simulink model "tfs"  (R2017b)
settings: Solver=FixedStepAuto  StartTime=0.0  StopTime=6  FixedStep=T  RelTol=1e-3  EnableMultiTasking=on
values from neighbouring files (symbols this model uses):
  d = [1 -2.638 2.284 -0.6455]    [EJECUTABLE.m]
  n = [0.01584 -0.03175 0.01594]    [EJECUTABLE.m]
undefined symbols (not defined in the file or in its folder): Controlador
settings Model: Creator=camal  LastModifiedBy=camal

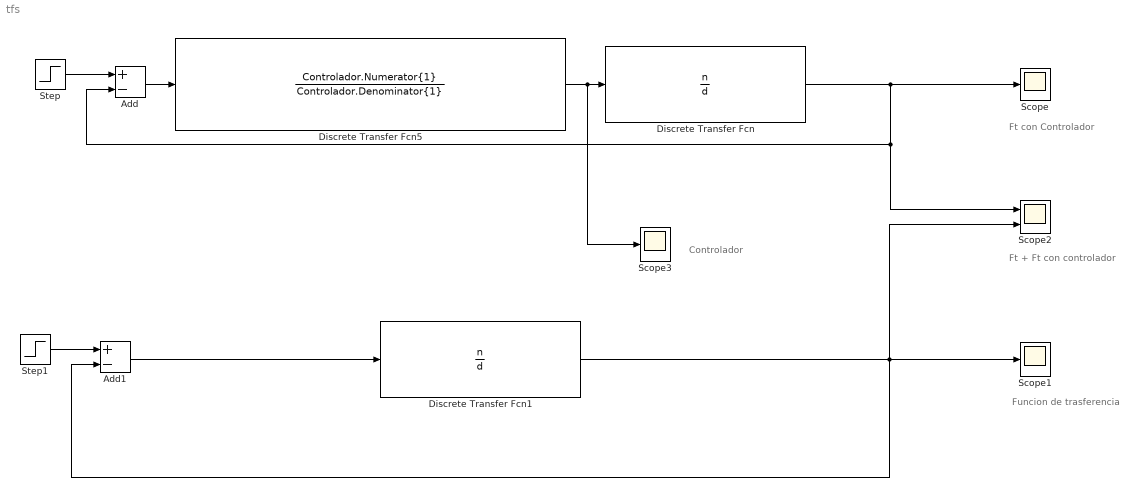
== system tfs ==
  note: Funcion de trasferencia
  note: Controlador
  note: Ft con Controlador
  note: Ft + Ft con controlador
  Add : Sum  Inputs=+-
  Add1 : Sum  Inputs=+-
  Discrete Transfer Fcn : DiscreteTransferFcn  Numerator=n  Denominator=d
  Discrete Transfer Fcn1 : DiscreteTransferFcn  Numerator=n  Denominator=d
  Discrete Transfer Fcn5 : DiscreteTransferFcn  Numerator=Controlador.Numerator{1}  Denominator=Controlador.Denominator{1}
  Scope : Scope
  Scope1 : Scope
  Scope2 : Scope  NumInputPorts=2
  Scope3 : Scope
  Step : Step  Time=0  SampleTime=0
  Step1 : Step  Time=0  SampleTime=0
  wires:
  Step/1 -> Add/1
  Step1/1 -> Add1/1
  Discrete Transfer Fcn1/1 -> Scope2/2, Scope1/1, Add1/2
  Add/1 -> Discrete Transfer Fcn5/1
  Discrete Transfer Fcn5/1 -> Scope3/1, Discrete Transfer Fcn/1
  Discrete Transfer Fcn/1 -> Scope/1, Add/2, Scope2/1
  Add1/1 -> Discrete Transfer Fcn1/1
